simulink model "test_pid_exact_3"  (R2021a)
settings: Solver=VariableStepAuto  StartTime=0.0  StopTime=2000  FixedStep=10  RelTol=1e-3
StopFcn:
  | out1=out;
values from neighbouring files (symbols this model uses):
  Force_Vectors = [Force_Vectors;normal_vector]    [ellip_force_test.m]    (also in initial_sim.m = Force_Vectors'; initial_sim2.m = Force_Vectors'; multi_sim.m = Force_Vectors'; multi_sim2.m = Force_Vectors')
  Km_d = inputArg(2)    [cost_pwpf_dis.m]
  max_f = 100000    [initial_sim.m]    (also in initial_sim2.m = 10)
  max_F_available = max_F_available*0.7    [initial_sim.m]    (also in initial_sim2.m)
  max_M_available = max_M_available*0.7    [initial_sim.m]    (also in initial_sim2.m; multi_sim.m; multi_sim2.m)
  mee_0 = oe2mee([a_0 e_0 incl_0 omega_0 RA_0 theta_0],p.mu)'    [Sample_OT.m]    (also in initial_sim.m = oe2mee(oe_0,params.mu)'; initial_sim2.m = oe2mee(oe_0,params.mu))
  Moment_Vectors = [Moment_Vectors;cross([x y z],normal_vector)]    [ellip_force_test.m]    (also in initial_sim.m = Moment_Vectors'; initial_sim2.m = Moment_Vectors'; multi_sim.m = Moment_Vectors'; multi_sim2.m = Moment_Vectors')
  N_sat = length(azimuths)    [ellip_force_test.m]    (also in initial_sim.m = 30; initial_sim2.m = 25; multi_sim.m = sim_data.N_sat; multi_sim2.m = sim_data.N_sat)
  out = (1+u).*cost_repo_limt.*(cost_repo).^2    [cost.m]    (also in cost2.m)
  params = 0    [Combo_OT.m]
  scale = length_real/(max(x)-min(x))    [model3d_maker.m]
  Tm_d = inputArg(1)    [cost_pwpf_dis.m]
  u_off = inputArg(4)    [cost_pwpf.m]    (also in cost_pwpf_dis.m)
  u_on = h+u_off    [cost_pwpf.m]    (also in cost_pwpf_dis.m)
undefined symbols (not defined in the file or in its folder): c_rad2deg, min_on_off_time, sample_time
libraries: pid_lib x8, simulink x3, shared6dof x1
settings Model: Creator=Mehdi  LastModifiedBy=Mehdi
settings SolverCC: ZeroCrossAlgorithm=Adaptive  AlgebraicLoopSolver=TrustRegion
settings DebuggingCC: IgnoredZcDiagnostic=none  SFMachineParentedDataDiag=warning

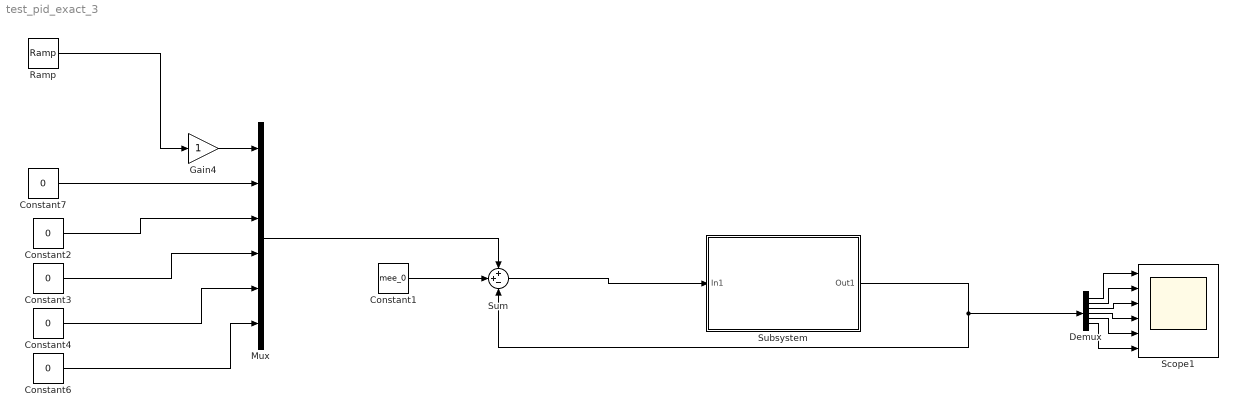
== system test_pid_exact_3 ==
  Constant1 : Constant  Value=mee_0
  Constant{2..4,6..7} (5 alike) : Constant  Value=0
  Demux : Demux  Outputs=6
  Gain4 : Gain
  Mux : Mux  Inputs=6
  Ramp : simulink/Sources/Ramp  slope=-40  start=1  InitialOutput=0
  Scope1 : Scope  NumInputPorts=6
  Subsystem : Subsystem
  Sum : Sum  Inputs=++-
  wires:
  Subsystem/1(Out1) -> Sum/3, Demux/1
  Demux/5 -> Scope1/5
  Demux/4 -> Scope1/4
  Demux/6 -> Scope1/6
  Demux/3 -> Scope1/3
  Demux/2 -> Scope1/2
  Demux/1 -> Scope1/1
  Constant1/1 -> Sum/2
  Constant7/1 -> Mux/2
  Constant2/1 -> Mux/3
  Constant3/1 -> Mux/4
  Constant4/1 -> Mux/5
  Sum/1 -> Subsystem/1(In1)
  Mux/1 -> Sum/1
  Constant6/1 -> Mux/6
  Ramp/1 -> Gain4/1
  Gain4/1 -> Mux/1

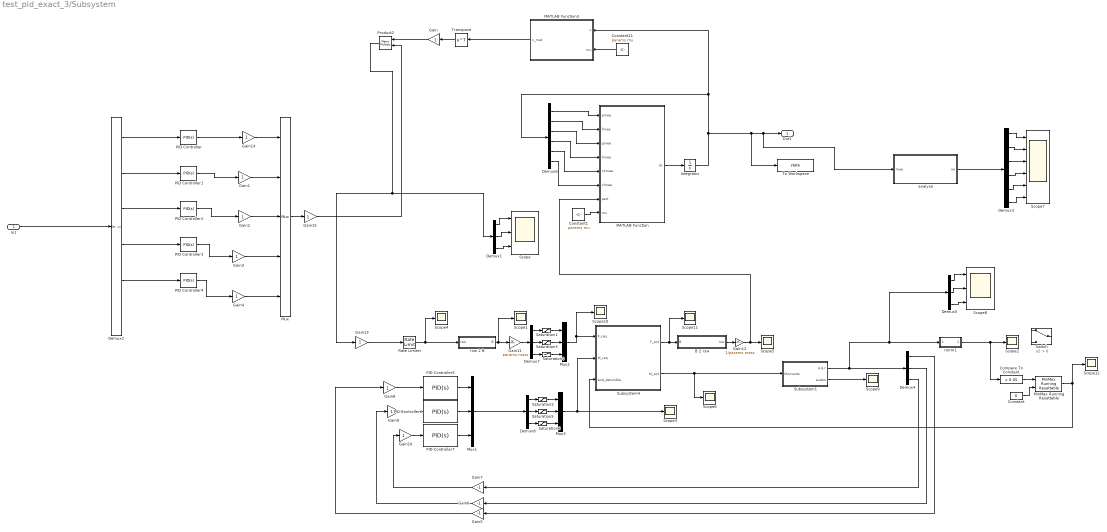
== system test_pid_exact_3/Subsystem ==
  In1 : Inport
  B 2 rsw : Subsystem
  Compare To Constant : simulink/Logic and Bit Operations/Compare To Constant  relop=<  const=0.05  OutDataTypeStr=boolean
  Constant : Constant  Value=0
  Constant1 : Constant  Value=params.mu
  Constant11 : Constant  Value=params.mu
  Demux{1,4..5,7..8} (5 alike) : Demux  Outputs=3
  Demux2 : Demux  Outputs=6
  Demux3 : Demux  Outputs=6
  Demux6 : Demux  Outputs=6
  Gain{,1..4,8..10,13..15} (11 alike) : Gain
  Gain11 : Gain  Gain=params.mass
  Gain12 : Gain  Gain=1/params.mass
  Gain5 : Gain  Gain=-1
  Gain6 : Gain  Gain=-1
  Gain7 : Gain  Gain=-1
  Integrator : Integrator  InitialCondition=mee_0
  MATLAB Function : MATLAB Function  TreatAsAtomicUnit=on
  MATLAB Function3 : MATLAB Function  TreatAsAtomicUnit=on
  MinMax Running Resettable : simulink/Math Operations/MinMax Running Resettable  Function=max  vinit=0.0
  Mux : Mux  Inputs=5
  Mux1 : Mux  Inputs=3
  Mux2 : Mux  Inputs=3
  Mux3 : Mux  Inputs=3
  PID Controller : pid_lib/PID Controller  Controller=PID  Form=Parallel  TimeDomain=Continuous-time  UseExternalTs=off  SampleTime=-1  IntegratorMethod=Forward Euler  FilterMethod=Forward Euler  ControllerParametersSource=internal  P=7.46892494212969e-17  I=7.69051114073229e-19  D=-6.40319929036286e-17  UseFilter=on  N=1.16643643332651  TunerSelectOption=Transfer Function Based (PID Tuner App)  InitialConditionSource=internal  InitialConditionForIntegrator=0  InitialConditionForFilter=0  DifferentiatorICPrevScaledInput=0  ExternalReset=none  TrackingMode=off  Kt=1  LimitOutput=off  SatLimitsSource=internal  UpperSaturationLimit=inf  LowerSaturationLimit=-inf  LinearizeAsGain=on  AntiWindupMode=none  Kb=1  POutMin=[]  POutMax=[]  IOutMin=[]  IOutMax=[]  DOutMin=[]  DOutMax=[]  NOutMin=[]  NOutMax=[]  SumOutMin=[]  SumOutMax=[]  SaturationOutMin=[]  SaturationOutMax=[]  PParamMin=[]  PParamMax=[]  IParamMin=[]  IParamMax=[]  DParamMin=[]  DParamMax=[]  NParamMin=[]  NParamMax=[]  KbParamMin=[]  KbParamMax=[]  KtParamMin=[]  KtParamMax=[]  KbOutMin=[]  KbOutMax=[]  KtOutMin=[]  KtOutMax=[]  IntegratorOutMin=[]  IntegratorOutMax=[]  FilterOutMin=[]  FilterOutMax=[]  SumI1OutMin=[]  SumI1OutMax=[]  SumI2OutMin=[]  SumI2OutMax=[]  SumI3OutMin=[]  SumI3OutMax=[]  SumI4OutMin=[]  SumI4OutMax=[]  SumDOutMin=[]  SumDOutMax=[]  DifferentiatorOutMin=[]  DifferentiatorOutMax=[]  FilterDiffOutCoefMin=[]  FilterDiffOutCoefMax=[]  ReciprocalOutMin=[]  ReciprocalOutMax=[]  SumDenOutMin=[]  SumDenOutMax=[]  SumNumOutMin=[]  SumNumOutMax=[]  DivideOutMin=[]  DivideOutMax=[]  UdiffTsProdOutMin=[]  UdiffTsProdOutMax=[]  NTsProdOutMin=[]  NTsProdOutMax=[]  UintegralTsProdOutMin=[]  UintegralTsProdOutMax=[]  UngainTsProdOutMin=[]  UngainTsProdOutMax=[]  IntegratorContinuousStateAttributes=''  IntegratorStateMustResolveToSignalObject=off  IntegratorRTWStateStorageClass=Auto  FilterContinuousStateAttributes=''  FilterStateMustResolveToSignalObject=off  FilterRTWStateStorageClass=Auto  ParallelPVariant=InternalParameters  IdealPVariant=Disabled  IVariant=InternalParameters  DVariant=InternalParameters  IntegratorVariant=Continuous  SatVariant=Disabled  AWVariant=Passthrough  PCopyVariant=Disabled  TRVariant=Disabled  FdbkBlocksVariant=Forward  IdealPFdbkVariant=Disabled  SatFdbkVariant=Disabled  DerivativeFilterVariant=ContFilter  NVariant=InternalParameters  NCopyVariant=Disabled  FilterICVariant=InternalICsFilter  IntegratorICVariant=InternalICs  ExternalResetVariant=Disabled  TRSumVariant=Passthrough  SumFdbkVariant=Disabled  SumVariant=Sum_PID  TsampFilterVariant=InternalTs  TsampNgainVariant=Passthrough  TsampIntegralVariant=Passthrough  ExternalSaturationOutDataTypeStr=Inherit: Same as second input
  PID Controller1 : pid_lib/PID Controller  Controller=PID  Form=Parallel  TimeDomain=Continuous-time  UseExternalTs=off  SampleTime=-1  IntegratorMethod=Forward Euler  FilterMethod=Forward Euler  ControllerParametersSource=internal  P=0.0771610720825314  I=1.00385329612141e-05  D=-57.2451341733765  UseFilter=on  N=0.000145942090581238  TunerSelectOption=Transfer Function Based (PID Tuner App)  InitialConditionSource=internal  InitialConditionForIntegrator=0  InitialConditionForFilter=0  DifferentiatorICPrevScaledInput=0  ExternalReset=none  TrackingMode=off  Kt=1  LimitOutput=off  SatLimitsSource=internal  UpperSaturationLimit=inf  LowerSaturationLimit=-inf  LinearizeAsGain=on  AntiWindupMode=none  Kb=1  POutMin=[]  POutMax=[]  IOutMin=[]  IOutMax=[]  DOutMin=[]  DOutMax=[]  NOutMin=[]  NOutMax=[]  SumOutMin=[]  SumOutMax=[]  SaturationOutMin=[]  SaturationOutMax=[]  PParamMin=[]  PParamMax=[]  IParamMin=[]  IParamMax=[]  DParamMin=[]  DParamMax=[]  NParamMin=[]  NParamMax=[]  KbParamMin=[]  KbParamMax=[]  KtParamMin=[]  KtParamMax=[]  KbOutMin=[]  KbOutMax=[]  KtOutMin=[]  KtOutMax=[]  IntegratorOutMin=[]  IntegratorOutMax=[]  FilterOutMin=[]  FilterOutMax=[]  SumI1OutMin=[]  SumI1OutMax=[]  SumI2OutMin=[]  SumI2OutMax=[]  SumI3OutMin=[]  SumI3OutMax=[]  SumI4OutMin=[]  SumI4OutMax=[]  SumDOutMin=[]  SumDOutMax=[]  DifferentiatorOutMin=[]  DifferentiatorOutMax=[]  FilterDiffOutCoefMin=[]  FilterDiffOutCoefMax=[]  ReciprocalOutMin=[]  ReciprocalOutMax=[]  SumDenOutMin=[]  SumDenOutMax=[]  SumNumOutMin=[]  SumNumOutMax=[]  DivideOutMin=[]  DivideOutMax=[]  UdiffTsProdOutMin=[]  UdiffTsProdOutMax=[]  NTsProdOutMin=[]  NTsProdOutMax=[]  UintegralTsProdOutMin=[]  UintegralTsProdOutMax=[]  UngainTsProdOutMin=[]  UngainTsProdOutMax=[]  IntegratorContinuousStateAttributes=''  IntegratorStateMustResolveToSignalObject=off  IntegratorRTWStateStorageClass=Auto  FilterContinuousStateAttributes=''  FilterStateMustResolveToSignalObject=off  FilterRTWStateStorageClass=Auto  ParallelPVariant=InternalParameters  IdealPVariant=Disabled  IVariant=InternalParameters  DVariant=InternalParameters  IntegratorVariant=Continuous  SatVariant=Disabled  AWVariant=Passthrough  PCopyVariant=Disabled  TRVariant=Disabled  FdbkBlocksVariant=Forward  IdealPFdbkVariant=Disabled  SatFdbkVariant=Disabled  DerivativeFilterVariant=ContFilter  NVariant=InternalParameters  NCopyVariant=Disabled  FilterICVariant=InternalICsFilter  IntegratorICVariant=InternalICs  ExternalResetVariant=Disabled  TRSumVariant=Passthrough  SumFdbkVariant=Disabled  SumVariant=Sum_PID  TsampFilterVariant=InternalTs  TsampNgainVariant=Passthrough  TsampIntegralVariant=Passthrough  ExternalSaturationOutDataTypeStr=Inherit: Same as second input
  PID Controller2 : pid_lib/PID Controller  Controller=PID  Form=Parallel  TimeDomain=Continuous-time  UseExternalTs=off  SampleTime=-1  IntegratorMethod=Forward Euler  FilterMethod=Forward Euler  ControllerParametersSource=internal  P=13.6496659854925  I=0.00798827574318409  D=-3629.49576294824  UseFilter=on  N=0.00260459411605955  TunerSelectOption=Transfer Function Based (PID Tuner App)  InitialConditionSource=internal  InitialConditionForIntegrator=0  InitialConditionForFilter=0  DifferentiatorICPrevScaledInput=0  ExternalReset=none  TrackingMode=off  Kt=1  LimitOutput=off  SatLimitsSource=internal  UpperSaturationLimit=inf  LowerSaturationLimit=-inf  LinearizeAsGain=on  AntiWindupMode=none  Kb=1  POutMin=[]  POutMax=[]  IOutMin=[]  IOutMax=[]  DOutMin=[]  DOutMax=[]  NOutMin=[]  NOutMax=[]  SumOutMin=[]  SumOutMax=[]  SaturationOutMin=[]  SaturationOutMax=[]  PParamMin=[]  PParamMax=[]  IParamMin=[]  IParamMax=[]  DParamMin=[]  DParamMax=[]  NParamMin=[]  NParamMax=[]  KbParamMin=[]  KbParamMax=[]  KtParamMin=[]  KtParamMax=[]  KbOutMin=[]  KbOutMax=[]  KtOutMin=[]  KtOutMax=[]  IntegratorOutMin=[]  IntegratorOutMax=[]  FilterOutMin=[]  FilterOutMax=[]  SumI1OutMin=[]  SumI1OutMax=[]  SumI2OutMin=[]  SumI2OutMax=[]  SumI3OutMin=[]  SumI3OutMax=[]  SumI4OutMin=[]  SumI4OutMax=[]  SumDOutMin=[]  SumDOutMax=[]  DifferentiatorOutMin=[]  DifferentiatorOutMax=[]  FilterDiffOutCoefMin=[]  FilterDiffOutCoefMax=[]  ReciprocalOutMin=[]  ReciprocalOutMax=[]  SumDenOutMin=[]  SumDenOutMax=[]  SumNumOutMin=[]  SumNumOutMax=[]  DivideOutMin=[]  DivideOutMax=[]  UdiffTsProdOutMin=[]  UdiffTsProdOutMax=[]  NTsProdOutMin=[]  NTsProdOutMax=[]  UintegralTsProdOutMin=[]  UintegralTsProdOutMax=[]  UngainTsProdOutMin=[]  UngainTsProdOutMax=[]  IntegratorContinuousStateAttributes=''  IntegratorStateMustResolveToSignalObject=off  IntegratorRTWStateStorageClass=Auto  FilterContinuousStateAttributes=''  FilterStateMustResolveToSignalObject=off  FilterRTWStateStorageClass=Auto  ParallelPVariant=InternalParameters  IdealPVariant=Disabled  IVariant=InternalParameters  DVariant=InternalParameters  IntegratorVariant=Continuous  SatVariant=Disabled  AWVariant=Passthrough  PCopyVariant=Disabled  TRVariant=Disabled  FdbkBlocksVariant=Forward  IdealPFdbkVariant=Disabled  SatFdbkVariant=Disabled  DerivativeFilterVariant=ContFilter  NVariant=InternalParameters  NCopyVariant=Disabled  FilterICVariant=InternalICsFilter  IntegratorICVariant=InternalICs  ExternalResetVariant=Disabled  TRSumVariant=Passthrough  SumFdbkVariant=Disabled  SumVariant=Sum_PID  TsampFilterVariant=InternalTs  TsampNgainVariant=Passthrough  TsampIntegralVariant=Passthrough  ExternalSaturationOutDataTypeStr=Inherit: Same as second input
  PID Controller3 : pid_lib/PID Controller  Controller=PID  Form=Parallel  TimeDomain=Continuous-time  UseExternalTs=off  SampleTime=-1  IntegratorMethod=Forward Euler  FilterMethod=Forward Euler  ControllerParametersSource=internal  P=1671.28261526635  I=9.96877148902592  D=-11671.5713850813  UseFilter=on  N=0.0760436593196284  TunerSelectOption=Transfer Function Based (PID Tuner App)  InitialConditionSource=internal  InitialConditionForIntegrator=0  InitialConditionForFilter=0  DifferentiatorICPrevScaledInput=0  ExternalReset=none  TrackingMode=off  Kt=1  LimitOutput=off  SatLimitsSource=internal  UpperSaturationLimit=inf  LowerSaturationLimit=-inf  LinearizeAsGain=on  AntiWindupMode=none  Kb=1  POutMin=[]  POutMax=[]  IOutMin=[]  IOutMax=[]  DOutMin=[]  DOutMax=[]  NOutMin=[]  NOutMax=[]  SumOutMin=[]  SumOutMax=[]  SaturationOutMin=[]  SaturationOutMax=[]  PParamMin=[]  PParamMax=[]  IParamMin=[]  IParamMax=[]  DParamMin=[]  DParamMax=[]  NParamMin=[]  NParamMax=[]  KbParamMin=[]  KbParamMax=[]  KtParamMin=[]  KtParamMax=[]  KbOutMin=[]  KbOutMax=[]  KtOutMin=[]  KtOutMax=[]  IntegratorOutMin=[]  IntegratorOutMax=[]  FilterOutMin=[]  FilterOutMax=[]  SumI1OutMin=[]  SumI1OutMax=[]  SumI2OutMin=[]  SumI2OutMax=[]  SumI3OutMin=[]  SumI3OutMax=[]  SumI4OutMin=[]  SumI4OutMax=[]  SumDOutMin=[]  SumDOutMax=[]  DifferentiatorOutMin=[]  DifferentiatorOutMax=[]  FilterDiffOutCoefMin=[]  FilterDiffOutCoefMax=[]  ReciprocalOutMin=[]  ReciprocalOutMax=[]  SumDenOutMin=[]  SumDenOutMax=[]  SumNumOutMin=[]  SumNumOutMax=[]  DivideOutMin=[]  DivideOutMax=[]  UdiffTsProdOutMin=[]  UdiffTsProdOutMax=[]  NTsProdOutMin=[]  NTsProdOutMax=[]  UintegralTsProdOutMin=[]  UintegralTsProdOutMax=[]  UngainTsProdOutMin=[]  UngainTsProdOutMax=[]  IntegratorContinuousStateAttributes=''  IntegratorStateMustResolveToSignalObject=off  IntegratorRTWStateStorageClass=Auto  FilterContinuousStateAttributes=''  FilterStateMustResolveToSignalObject=off  FilterRTWStateStorageClass=Auto  ParallelPVariant=InternalParameters  IdealPVariant=Disabled  IVariant=InternalParameters  DVariant=InternalParameters  IntegratorVariant=Continuous  SatVariant=Disabled  AWVariant=Passthrough  PCopyVariant=Disabled  TRVariant=Disabled  FdbkBlocksVariant=Forward  IdealPFdbkVariant=Disabled  SatFdbkVariant=Disabled  DerivativeFilterVariant=ContFilter  NVariant=InternalParameters  NCopyVariant=Disabled  FilterICVariant=InternalICsFilter  IntegratorICVariant=InternalICs  ExternalResetVariant=Disabled  TRSumVariant=Passthrough  SumFdbkVariant=Disabled  SumVariant=Sum_PID  TsampFilterVariant=InternalTs  TsampNgainVariant=Passthrough  TsampIntegralVariant=Passthrough  ExternalSaturationOutDataTypeStr=Inherit: Same as second input
  PID Controller4 : pid_lib/PID Controller  Controller=PID  Form=Parallel  TimeDomain=Continuous-time  UseExternalTs=off  SampleTime=-1  IntegratorMethod=Forward Euler  FilterMethod=Forward Euler  ControllerParametersSource=internal  P=479.365255304021  I=32.91768970317  D=214.700467675545  UseFilter=on  N=13.9469234742288  TunerSelectOption=Transfer Function Based (PID Tuner App)  InitialConditionSource=internal  InitialConditionForIntegrator=0  InitialConditionForFilter=0  DifferentiatorICPrevScaledInput=0  ExternalReset=none  TrackingMode=off  Kt=1  LimitOutput=off  SatLimitsSource=internal  UpperSaturationLimit=inf  LowerSaturationLimit=-inf  LinearizeAsGain=on  AntiWindupMode=none  Kb=1  POutMin=[]  POutMax=[]  IOutMin=[]  IOutMax=[]  DOutMin=[]  DOutMax=[]  NOutMin=[]  NOutMax=[]  SumOutMin=[]  SumOutMax=[]  SaturationOutMin=[]  SaturationOutMax=[]  PParamMin=[]  PParamMax=[]  IParamMin=[]  IParamMax=[]  DParamMin=[]  DParamMax=[]  NParamMin=[]  NParamMax=[]  KbParamMin=[]  KbParamMax=[]  KtParamMin=[]  KtParamMax=[]  KbOutMin=[]  KbOutMax=[]  KtOutMin=[]  KtOutMax=[]  IntegratorOutMin=[]  IntegratorOutMax=[]  FilterOutMin=[]  FilterOutMax=[]  SumI1OutMin=[]  SumI1OutMax=[]  SumI2OutMin=[]  SumI2OutMax=[]  SumI3OutMin=[]  SumI3OutMax=[]  SumI4OutMin=[]  SumI4OutMax=[]  SumDOutMin=[]  SumDOutMax=[]  DifferentiatorOutMin=[]  DifferentiatorOutMax=[]  FilterDiffOutCoefMin=[]  FilterDiffOutCoefMax=[]  ReciprocalOutMin=[]  ReciprocalOutMax=[]  SumDenOutMin=[]  SumDenOutMax=[]  SumNumOutMin=[]  SumNumOutMax=[]  DivideOutMin=[]  DivideOutMax=[]  UdiffTsProdOutMin=[]  UdiffTsProdOutMax=[]  NTsProdOutMin=[]  NTsProdOutMax=[]  UintegralTsProdOutMin=[]  UintegralTsProdOutMax=[]  UngainTsProdOutMin=[]  UngainTsProdOutMax=[]  IntegratorContinuousStateAttributes=''  IntegratorStateMustResolveToSignalObject=off  IntegratorRTWStateStorageClass=Auto  FilterContinuousStateAttributes=''  FilterStateMustResolveToSignalObject=off  FilterRTWStateStorageClass=Auto  ParallelPVariant=InternalParameters  IdealPVariant=Disabled  IVariant=InternalParameters  DVariant=InternalParameters  IntegratorVariant=Continuous  SatVariant=Disabled  AWVariant=Passthrough  PCopyVariant=Disabled  TRVariant=Disabled  FdbkBlocksVariant=Forward  IdealPFdbkVariant=Disabled  SatFdbkVariant=Disabled  DerivativeFilterVariant=ContFilter  NVariant=InternalParameters  NCopyVariant=Disabled  FilterICVariant=InternalICsFilter  IntegratorICVariant=InternalICs  ExternalResetVariant=Disabled  TRSumVariant=Passthrough  SumFdbkVariant=Disabled  SumVariant=Sum_PID  TsampFilterVariant=InternalTs  TsampNgainVariant=Passthrough  TsampIntegralVariant=Passthrough  ExternalSaturationOutDataTypeStr=Inherit: Same as second input
  PID Controller5 : pid_lib/PID Controller  Controller=PID  Form=Parallel  TimeDomain=Continuous-time  UseExternalTs=off  SampleTime=-1  IntegratorMethod=Forward Euler  FilterMethod=Forward Euler  ControllerParametersSource=internal  P=493.267124009933  I=0.0943532881280952  D=-103949.358808414  UseFilter=on  N=0.00172044274974478  TunerSelectOption=Transfer Function Based (PID Tuner App)  InitialConditionSource=internal  InitialConditionForIntegrator=0  InitialConditionForFilter=0  DifferentiatorICPrevScaledInput=0  ExternalReset=none  TrackingMode=off  Kt=1  LimitOutput=off  SatLimitsSource=internal  UpperSaturationLimit=inf  LowerSaturationLimit=-inf  LinearizeAsGain=on  AntiWindupMode=none  Kb=1  POutMin=[]  POutMax=[]  IOutMin=[]  IOutMax=[]  DOutMin=[]  DOutMax=[]  NOutMin=[]  NOutMax=[]  SumOutMin=[]  SumOutMax=[]  SaturationOutMin=[]  SaturationOutMax=[]  PParamMin=[]  PParamMax=[]  IParamMin=[]  IParamMax=[]  DParamMin=[]  DParamMax=[]  NParamMin=[]  NParamMax=[]  KbParamMin=[]  KbParamMax=[]  KtParamMin=[]  KtParamMax=[]  KbOutMin=[]  KbOutMax=[]  KtOutMin=[]  KtOutMax=[]  IntegratorOutMin=[]  IntegratorOutMax=[]  FilterOutMin=[]  FilterOutMax=[]  SumI1OutMin=[]  SumI1OutMax=[]  SumI2OutMin=[]  SumI2OutMax=[]  SumI3OutMin=[]  SumI3OutMax=[]  SumI4OutMin=[]  SumI4OutMax=[]  SumDOutMin=[]  SumDOutMax=[]  DifferentiatorOutMin=[]  DifferentiatorOutMax=[]  FilterDiffOutCoefMin=[]  FilterDiffOutCoefMax=[]  ReciprocalOutMin=[]  ReciprocalOutMax=[]  SumDenOutMin=[]  SumDenOutMax=[]  SumNumOutMin=[]  SumNumOutMax=[]  DivideOutMin=[]  DivideOutMax=[]  UdiffTsProdOutMin=[]  UdiffTsProdOutMax=[]  NTsProdOutMin=[]  NTsProdOutMax=[]  UintegralTsProdOutMin=[]  UintegralTsProdOutMax=[]  UngainTsProdOutMin=[]  UngainTsProdOutMax=[]  IntegratorContinuousStateAttributes=''  IntegratorStateMustResolveToSignalObject=off  IntegratorRTWStateStorageClass=Auto  FilterContinuousStateAttributes=''  FilterStateMustResolveToSignalObject=off  FilterRTWStateStorageClass=Auto  ParallelPVariant=InternalParameters  IdealPVariant=Disabled  IVariant=InternalParameters  DVariant=InternalParameters  IntegratorVariant=Continuous  SatVariant=Disabled  AWVariant=Passthrough  PCopyVariant=Disabled  TRVariant=Disabled  FdbkBlocksVariant=Forward  IdealPFdbkVariant=Disabled  SatFdbkVariant=Disabled  DerivativeFilterVariant=ContFilter  NVariant=InternalParameters  NCopyVariant=Disabled  FilterICVariant=InternalICsFilter  IntegratorICVariant=InternalICs  ExternalResetVariant=Disabled  TRSumVariant=Passthrough  SumFdbkVariant=Disabled  SumVariant=Sum_PID  TsampFilterVariant=InternalTs  TsampNgainVariant=Passthrough  TsampIntegralVariant=Passthrough  ExternalSaturationOutDataTypeStr=Inherit: Same as second input
  PID Controller6 : pid_lib/PID Controller  Controller=PID  Form=Parallel  TimeDomain=Continuous-time  UseExternalTs=off  SampleTime=-1  IntegratorMethod=Forward Euler  FilterMethod=Forward Euler  ControllerParametersSource=internal  P=493.267124009933  I=0.0943532881280952  D=-103949.358808414  UseFilter=on  N=0.00172044274974478  TunerSelectOption=Transfer Function Based (PID Tuner App)  InitialConditionSource=internal  InitialConditionForIntegrator=0  InitialConditionForFilter=0  DifferentiatorICPrevScaledInput=0  ExternalReset=none  TrackingMode=off  Kt=1  LimitOutput=off  SatLimitsSource=internal  UpperSaturationLimit=inf  LowerSaturationLimit=-inf  LinearizeAsGain=on  AntiWindupMode=none  Kb=1  POutMin=[]  POutMax=[]  IOutMin=[]  IOutMax=[]  DOutMin=[]  DOutMax=[]  NOutMin=[]  NOutMax=[]  SumOutMin=[]  SumOutMax=[]  SaturationOutMin=[]  SaturationOutMax=[]  PParamMin=[]  PParamMax=[]  IParamMin=[]  IParamMax=[]  DParamMin=[]  DParamMax=[]  NParamMin=[]  NParamMax=[]  KbParamMin=[]  KbParamMax=[]  KtParamMin=[]  KtParamMax=[]  KbOutMin=[]  KbOutMax=[]  KtOutMin=[]  KtOutMax=[]  IntegratorOutMin=[]  IntegratorOutMax=[]  FilterOutMin=[]  FilterOutMax=[]  SumI1OutMin=[]  SumI1OutMax=[]  SumI2OutMin=[]  SumI2OutMax=[]  SumI3OutMin=[]  SumI3OutMax=[]  SumI4OutMin=[]  SumI4OutMax=[]  SumDOutMin=[]  SumDOutMax=[]  DifferentiatorOutMin=[]  DifferentiatorOutMax=[]  FilterDiffOutCoefMin=[]  FilterDiffOutCoefMax=[]  ReciprocalOutMin=[]  ReciprocalOutMax=[]  SumDenOutMin=[]  SumDenOutMax=[]  SumNumOutMin=[]  SumNumOutMax=[]  DivideOutMin=[]  DivideOutMax=[]  UdiffTsProdOutMin=[]  UdiffTsProdOutMax=[]  NTsProdOutMin=[]  NTsProdOutMax=[]  UintegralTsProdOutMin=[]  UintegralTsProdOutMax=[]  UngainTsProdOutMin=[]  UngainTsProdOutMax=[]  IntegratorContinuousStateAttributes=''  IntegratorStateMustResolveToSignalObject=off  IntegratorRTWStateStorageClass=Auto  FilterContinuousStateAttributes=''  FilterStateMustResolveToSignalObject=off  FilterRTWStateStorageClass=Auto  ParallelPVariant=InternalParameters  IdealPVariant=Disabled  IVariant=InternalParameters  DVariant=InternalParameters  IntegratorVariant=Continuous  SatVariant=Disabled  AWVariant=Passthrough  PCopyVariant=Disabled  TRVariant=Disabled  FdbkBlocksVariant=Forward  IdealPFdbkVariant=Disabled  SatFdbkVariant=Disabled  DerivativeFilterVariant=ContFilter  NVariant=InternalParameters  NCopyVariant=Disabled  FilterICVariant=InternalICsFilter  IntegratorICVariant=InternalICs  ExternalResetVariant=Disabled  TRSumVariant=Passthrough  SumFdbkVariant=Disabled  SumVariant=Sum_PID  TsampFilterVariant=InternalTs  TsampNgainVariant=Passthrough  TsampIntegralVariant=Passthrough  ExternalSaturationOutDataTypeStr=Inherit: Same as second input
  PID Controller7 : pid_lib/PID Controller  Controller=PID  Form=Parallel  TimeDomain=Continuous-time  UseExternalTs=off  SampleTime=-1  IntegratorMethod=Forward Euler  FilterMethod=Forward Euler  ControllerParametersSource=internal  P=493.267124009933  I=0.0943532881280952  D=-103949.358808414  UseFilter=on  N=0.00172044274974478  TunerSelectOption=Transfer Function Based (PID Tuner App)  InitialConditionSource=internal  InitialConditionForIntegrator=0  InitialConditionForFilter=0  DifferentiatorICPrevScaledInput=0  ExternalReset=none  TrackingMode=off  Kt=1  LimitOutput=off  SatLimitsSource=internal  UpperSaturationLimit=inf  LowerSaturationLimit=-inf  LinearizeAsGain=on  AntiWindupMode=none  Kb=1  POutMin=[]  POutMax=[]  IOutMin=[]  IOutMax=[]  DOutMin=[]  DOutMax=[]  NOutMin=[]  NOutMax=[]  SumOutMin=[]  SumOutMax=[]  SaturationOutMin=[]  SaturationOutMax=[]  PParamMin=[]  PParamMax=[]  IParamMin=[]  IParamMax=[]  DParamMin=[]  DParamMax=[]  NParamMin=[]  NParamMax=[]  KbParamMin=[]  KbParamMax=[]  KtParamMin=[]  KtParamMax=[]  KbOutMin=[]  KbOutMax=[]  KtOutMin=[]  KtOutMax=[]  IntegratorOutMin=[]  IntegratorOutMax=[]  FilterOutMin=[]  FilterOutMax=[]  SumI1OutMin=[]  SumI1OutMax=[]  SumI2OutMin=[]  SumI2OutMax=[]  SumI3OutMin=[]  SumI3OutMax=[]  SumI4OutMin=[]  SumI4OutMax=[]  SumDOutMin=[]  SumDOutMax=[]  DifferentiatorOutMin=[]  DifferentiatorOutMax=[]  FilterDiffOutCoefMin=[]  FilterDiffOutCoefMax=[]  ReciprocalOutMin=[]  ReciprocalOutMax=[]  SumDenOutMin=[]  SumDenOutMax=[]  SumNumOutMin=[]  SumNumOutMax=[]  DivideOutMin=[]  DivideOutMax=[]  UdiffTsProdOutMin=[]  UdiffTsProdOutMax=[]  NTsProdOutMin=[]  NTsProdOutMax=[]  UintegralTsProdOutMin=[]  UintegralTsProdOutMax=[]  UngainTsProdOutMin=[]  UngainTsProdOutMax=[]  IntegratorContinuousStateAttributes=''  IntegratorStateMustResolveToSignalObject=off  IntegratorRTWStateStorageClass=Auto  FilterContinuousStateAttributes=''  FilterStateMustResolveToSignalObject=off  FilterRTWStateStorageClass=Auto  ParallelPVariant=InternalParameters  IdealPVariant=Disabled  IVariant=InternalParameters  DVariant=InternalParameters  IntegratorVariant=Continuous  SatVariant=Disabled  AWVariant=Passthrough  PCopyVariant=Disabled  TRVariant=Disabled  FdbkBlocksVariant=Forward  IdealPFdbkVariant=Disabled  SatFdbkVariant=Disabled  DerivativeFilterVariant=ContFilter  NVariant=InternalParameters  NCopyVariant=Disabled  FilterICVariant=InternalICsFilter  IntegratorICVariant=InternalICs  ExternalResetVariant=Disabled  TRSumVariant=Passthrough  SumFdbkVariant=Disabled  SumVariant=Sum_PID  TsampFilterVariant=InternalTs  TsampNgainVariant=Passthrough  TsampIntegralVariant=Passthrough  ExternalSaturationOutDataTypeStr=Inherit: Same as second input
  Product2 : Product  Multiplication=Matrix(*)
  Rate Limiter : RateLimiter  RisingSlewLimit=1e-4  FallingSlewLimit=-1e-4  SampleTimeMode=inherited
  Saturation1 : Saturate  UpperLimit=max_F_available(1,1)  LowerLimit=max_F_available(1,2)
  Saturation2 : Saturate  UpperLimit=max_M_available(1,1)  LowerLimit=max_M_available(1,2)
  Saturation3 : Saturate  UpperLimit=max_F_available(2,1)  LowerLimit=max_F_available(2,2)
  Saturation4 : Saturate  UpperLimit=max_F_available(3,1)  LowerLimit=max_F_available(3,2)
  Saturation5 : Saturate  UpperLimit=max_M_available(2,1)  LowerLimit=max_M_available(2,2)
  Saturation6 : Saturate  UpperLimit=max_M_available(3,1)  LowerLimit=max_M_available(3,2)
  Scope : Scope  NumInputPorts=3
  Scope{1..6,9..12} (10 alike) : Scope
  Scope7 : Scope  NumInputPorts=6
  Scope8 : Scope  NumInputPorts=3
  Subsystem1 : Subsystem
  Subsystem4 : Subsystem
  Switch : Switch  Criteria=u2 > Threshold
  To Workspace : ToWorkspace  VariableName=state  SaveFormat=Timeseries  SampleTime=-1
  Transpose : Math  Operator=transpose  SaturateOnIntegerOverflow=on
  analyse : Subsystem
  norm1 : Subsystem
  rsw 2 B : Subsystem
  Out1 : Outport
  wires:
  Demux6/2 -> MATLAB Function/2(fmee)
  Demux6/1 -> MATLAB Function/1(pmee)
  Demux6/3 -> MATLAB Function/3(gmee)
  Demux6/4 -> MATLAB Function/4(hmee)
  Demux6/5 -> MATLAB Function/5(xkmee)
  Demux6/6 -> MATLAB Function/6(xlmee)
  MATLAB Function/1(dx) -> Integrator/1
  Constant11/1 -> MATLAB Function3/2(mu)
  MATLAB Function3/1(c_mat) -> Transpose/1
  Constant1/1 -> MATLAB Function/8(mu)
  Transpose/1 -> Gain/1
  Gain/1 -> Product2/1
  Demux1/3 -> Scope/3
  Demux1/2 -> Scope/2
  Demux1/1 -> Scope/1
  Demux2/4 -> PID Controller3/1
  Demux2/3 -> PID Controller2/1
  Demux2/5 -> PID Controller4/1
  Demux2/2 -> PID Controller1/1
  Demux2/1 -> PID Controller/1
  In1/1 -> Demux2/1
  Mux/1 -> Gain15/1
  PID Controller/1 -> Gain14/1
  PID Controller1/1 -> Gain1/1
  PID Controller2/1 -> Gain2/1
  PID Controller3/1 -> Gain3/1
  PID Controller4/1 -> Gain4/1
  Gain1/1 -> Mux/2
  Gain2/1 -> Mux/3
  Gain3/1 -> Mux/4
  Gain4/1 -> Mux/5
  Subsystem4/2(M_act) -> Subsystem1/1(Moments), Scope6/1
  Product2/1 -> Gain13/1, Demux1/1
  Demux3/6 -> Scope7/6
  Demux3/1 -> Scope7/1
  Demux3/2 -> Scope7/2
  Demux3/3 -> Scope7/3
  Demux3/4 -> Scope7/4
  Demux3/5 -> Scope7/5
  Integrator/1 -> To Workspace/1, analyse/1(mee), Out1/1, Demux6/1, MATLAB Function3/1(x)
  analyse/1(oe) -> Demux3/1
  Rate Limiter/1 -> rsw 2 B/1(rsw), Scope4/1
  Subsystem4/1(F_act) -> Scope11/1, B 2 rsw/1(B)
  B 2 rsw/1(rsw) -> Gain12/1
  rsw 2 B/1(B) -> Gain11/1, Scope1/1
  Gain8/1 -> PID Controller5/1
  Gain9/1 -> PID Controller6/1
  PID Controller7/1 -> Mux1/3
  Gain7/1 -> Gain10/1
  Demux4/1 -> Gain5/1
  Gain6/1 -> Gain9/1
  Subsystem1/2(eulers) -> Scope9/1
  Demux4/2 -> Gain6/1
  PID Controller5/1 -> Mux1/1
  Demux4/3 -> Gain7/1
  Gain10/1 -> PID Controller7/1
  Gain5/1 -> Gain8/1
  PID Controller6/1 -> Mux1/2
  norm1/1(Out1) -> Scope2/1, Compare To Constant/1
  Subsystem1/1(p,q,r) -> Demux5/1, norm1/1(p,q,r), Demux4/1
  Demux5/1 -> Scope8/1
  Demux5/3 -> Scope8/3
  Demux5/2 -> Scope8/2
  Mux3/1 -> Subsystem4/2(M_req), Scope3/1
  Demux7/1 -> Saturation1/1
  Demux7/2 -> Saturation3/1
  Demux7/3 -> Saturation4/1
  Saturation1/1 -> Mux2/1
  Saturation3/1 -> Mux2/2
  Saturation4/1 -> Mux2/3
  Mux2/1 -> Scope10/1, Subsystem4/1(F_req)
  Demux8/1 -> Saturation2/1
  Demux8/3 -> Saturation6/1
  Saturation6/1 -> Mux3/3
  Saturation5/1 -> Mux3/2
  Demux8/2 -> Saturation5/1
  Saturation2/1 -> Mux3/1
  Mux1/1 -> Demux8/1
  Gain11/1 -> Demux7/1
  Gain12/1 -> Scope5/1, MATLAB Function/7(pert)
  Gain13/1 -> Rate Limiter/1
  Gain14/1 -> Mux/1
  Gain15/1 -> Product2/2
  MinMax Running Resettable/1 -> Scope12/1, Subsystem4/3(end_detumble)
  Compare To Constant/1 -> MinMax Running Resettable/1
  Constant/1 -> MinMax Running Resettable/2

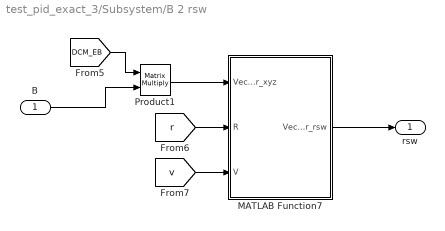
== system test_pid_exact_3/Subsystem/B 2 rsw ==
  B : Inport
  MATLAB Function7 : MATLAB Function  TreatAsAtomicUnit=on
  Product1 : Product  Multiplication=Matrix(*)
  rsw : Outport
  wires:
  Product1/1 -> MATLAB Function7/1(Vector_xyz)
  [v] -> MATLAB Function7/3(V)
  [DCM_EB] -> Product1/1
  [r] -> MATLAB Function7/2(R)
  B/1 -> Product1/2
  MATLAB Function7/1(Vector_rsw) -> rsw/1

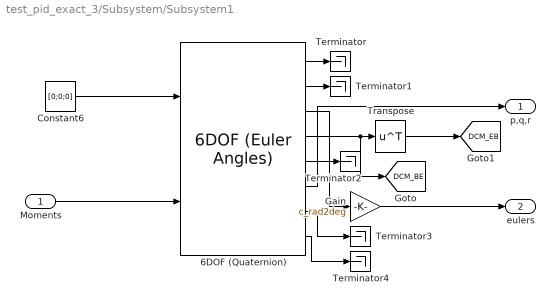
== system test_pid_exact_3/Subsystem/Subsystem1 ==
  Moments : Inport
  6DOF (Quaternion) : shared6dof/6DOF (Euler Angles)  units=Metric (MKS)  mtype=Fixed  rep=Quaternion  xme_0=[0 0 0]  Vm_0=[0 0 0]  eul_0=eul_0  pm_0=pqr_0  mass_0=1.0  mass_e=0.5  mass_f=2.0  inertia=params.Inertia  inertia_e=eye(3)  inertia_f=2*eye(3)  k_quat=1.0  vre_flag=on  abi_flag=off  aMode=0  xme_statename=''  Vm_statename=''  eul_statename=''  quat_statename=''  pm_statename=''  mass_statename=''
      settings: SourceProductBaseCode=AE,PW,DR,MT,UV,VE
  Constant6 : Constant  Value=[0;0;0]
  Gain : Gain  Gain=c_rad2deg
  Terminator{,1..4} (5 alike) : Terminator
  Transpose : Math  Operator=transpose  SaturateOnIntegerOverflow=on
  p,q,r : Outport
  eulers : Outport  Port=2
  tag scope: DCM_BE=global, DCM_EB=global
  wires:
  6DOF (Quaternion)/7 -> Terminator3/1
  Constant6/1 -> 6DOF (Quaternion)/1
  6DOF (Quaternion)/3 -> Gain/1
  6DOF (Quaternion)/1 -> Terminator/1
  6DOF (Quaternion)/6 -> p,q,r/1
  6DOF (Quaternion)/5 -> Terminator2/1
  6DOF (Quaternion)/2 -> Terminator1/1
  Gain/1 -> eulers/1
  6DOF (Quaternion)/4 -> [DCM_BE], Transpose/1
  6DOF (Quaternion)/8 -> Terminator4/1
  Moments/1 -> 6DOF (Quaternion)/2
  Transpose/1 -> [DCM_EB]

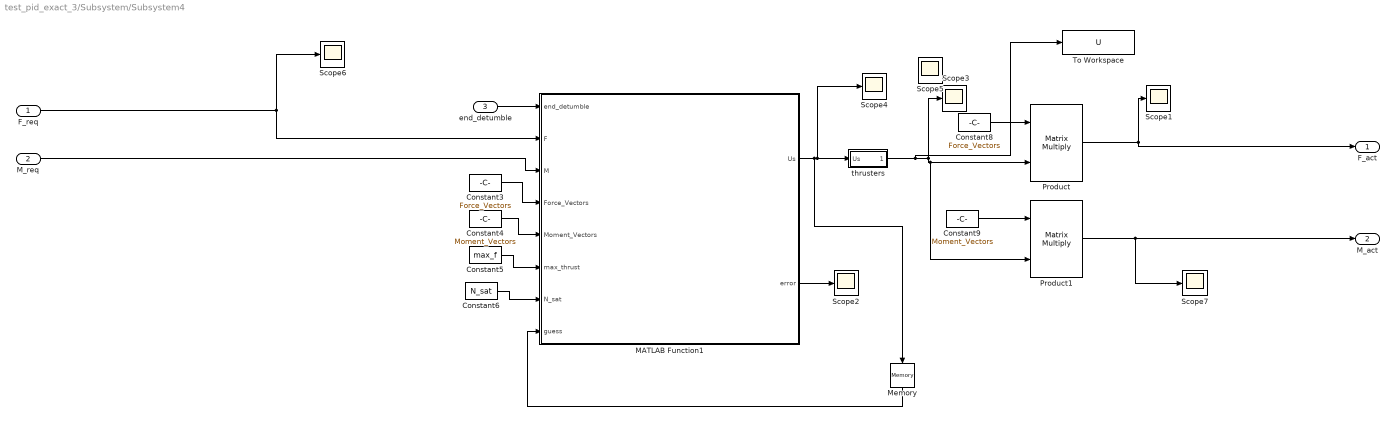
== system test_pid_exact_3/Subsystem/Subsystem4 ==
  F_req : Inport
  M_req : Inport  Port=2
  end_detumble : Inport  Port=3
  Constant3 : Constant  Value=Force_Vectors
  Constant4 : Constant  Value=Moment_Vectors
  Constant5 : Constant  Value=max_f
  Constant6 : Constant  Value=N_sat
  Constant8 : Constant  Value=Force_Vectors
  Constant9 : Constant  Value=Moment_Vectors
  MATLAB Function1 : MATLAB Function  TreatAsAtomicUnit=on
  Memory : Memory  InitialCondition=zeros(N_sat,1)
  Product : Product  Multiplication=Matrix(*)
  Product1 : Product  Multiplication=Matrix(*)
  Scope{1..7} (7 alike) : Scope
  To Workspace : ToWorkspace  VariableName=U  SaveFormat=Timeseries  SampleTime=-1
  thrusters : Subsystem
  F_act : Outport
  M_act : Outport  Port=2
  wires:
  Constant6/1 -> MATLAB Function1/7(N_sat)
  Constant9/1 -> Product1/1
  Memory/1 -> MATLAB Function1/8(guess)
  MATLAB Function1/2(error) -> Scope2/1
  Constant3/1 -> MATLAB Function1/4(Force_Vectors)
  Constant4/1 -> MATLAB Function1/5(Moment_Vectors)
  Product1/1 -> Scope7/1, M_act/1
  Constant8/1 -> Product/1
  Constant5/1 -> MATLAB Function1/6(max_thrust)
  F_req/1 -> MATLAB Function1/2(F), Scope6/1
  M_req/1 -> MATLAB Function1/3(M)
  Product/1 -> F_act/1, Scope1/1
  end_detumble/1 -> MATLAB Function1/1(end_detumble)
  MATLAB Function1/1(Us) -> thrusters/1(Us), Scope4/1, Memory/1
  thrusters/1(U_act) -> To Workspace/1, Product/2, Product1/2, Scope3/1

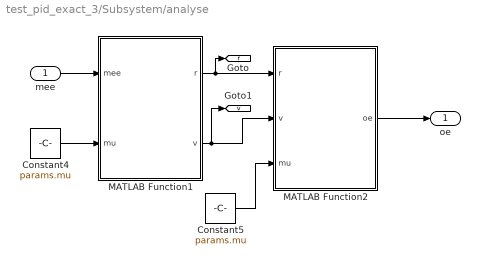
== system test_pid_exact_3/Subsystem/analyse ==
  mee : Inport
  Constant4 : Constant  Value=params.mu
  Constant5 : Constant  Value=params.mu
  MATLAB Function1 : MATLAB Function  TreatAsAtomicUnit=on
  MATLAB Function2 : MATLAB Function  TreatAsAtomicUnit=on
  oe : Outport
  tag scope: r=global, v=global
  wires:
  Constant5/1 -> MATLAB Function2/3(mu)
  Constant4/1 -> MATLAB Function1/2(mu)
  MATLAB Function1/1(r) -> [r], MATLAB Function2/1(r)
  MATLAB Function1/2(v) -> [v], MATLAB Function2/2(v)
  MATLAB Function2/1(oe) -> oe/1
  mee/1 -> MATLAB Function1/1(mee)

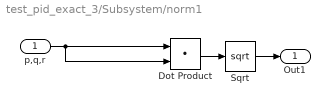
== system test_pid_exact_3/Subsystem/norm1 ==
  p,q,r : Inport
  Dot Product : DotProduct  InputSameDT=on  OutDataTypeStr=Inherit: Inherit via internal rule
  Sqrt : Sqrt  OutputSignalType=real  SaturateOnIntegerOverflow=on
  Out1 : Outport
  wires:
  Dot Product/1 -> Sqrt/1
  p,q,r/1 -> Dot Product/1, Dot Product/2
  Sqrt/1 -> Out1/1

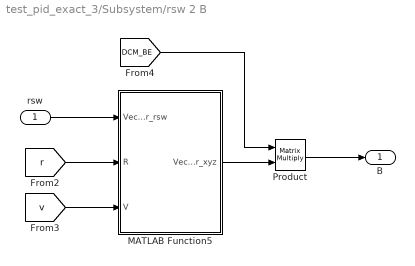
== system test_pid_exact_3/Subsystem/rsw 2 B ==
  rsw : Inport
  MATLAB Function5 : MATLAB Function  TreatAsAtomicUnit=on
  Product : Product  Multiplication=Matrix(*)
  B : Outport
  wires:
  [DCM_BE] -> Product/1
  rsw/1 -> MATLAB Function5/1(Vector_rsw)
  MATLAB Function5/1(Vector_xyz) -> Product/2
  [v] -> MATLAB Function5/3(V)
  [r] -> MATLAB Function5/2(R)
  Product/1 -> B/1

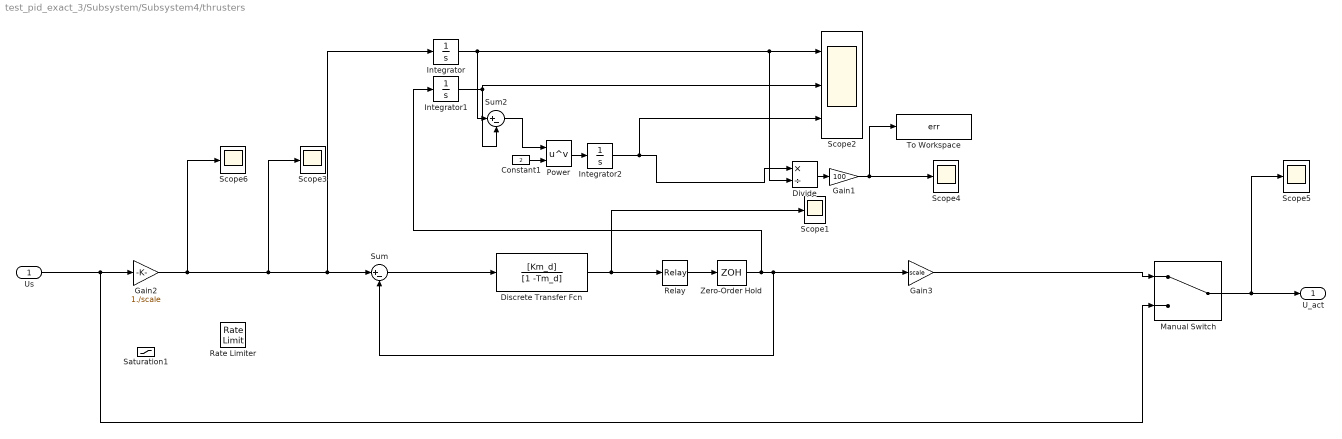
== system test_pid_exact_3/Subsystem/Subsystem4/thrusters ==
  Us : Inport
  Constant1 : Constant  Value=2  VectorParams1D=off
  Discrete Transfer Fcn : DiscreteTransferFcn  Numerator=[Km_d]  Denominator=[1 -Tm_d]  SampleTime=sample_time
  Divide : Product  Inputs=*/
  Gain1 : Gain  Gain=100
  Gain2 : Gain  Gain=1./scale
  Gain3 : Gain  Gain=scale
  Integrator : Integrator
  Integrator1 : Integrator
  Integrator2 : Integrator
  Manual Switch : ManualSwitch
  Power : Math  Operator=pow  SaturateOnIntegerOverflow=on
  Rate Limiter : RateLimiter  RisingSlewLimit=1e-4  FallingSlewLimit=-1e-4  SampleTimeMode=inherited
  Relay : Relay  OnSwitchValue=u_on  OffSwitchValue=u_off  OnOutputValue=Thrust_digital
  Saturation1 : Saturate  UpperLimit=max_f  LowerLimit=0
  Scope{1,3..6} (5 alike) : Scope
  Scope2 : Scope  NumInputPorts=3
  Sum : Sum  Inputs=|+-
  Sum2 : Sum  Inputs=|+-
  To Workspace : ToWorkspace  VariableName=err  SaveFormat=Timeseries  SampleTime=-1
      settings: MaxDataPoints=1
  Zero-Order Hold : ZeroOrderHold  SampleTime=min_on_off_time
  U_act : Outport
  wires:
  Manual Switch/1 -> Scope5/1, U_act/1
  Gain3/1 -> Manual Switch/1
  Divide/1 -> Gain1/1
  Zero-Order Hold/1 -> Integrator1/1, Sum/2, Gain3/1
  Sum/1 -> Discrete Transfer Fcn/1
  Gain1/1 -> To Workspace/1, Scope4/1
  Relay/1 -> Zero-Order Hold/1
  Constant1/1 -> Power/2
  Integrator1/1 -> Sum2/2, Scope2/2
  Discrete Transfer Fcn/1 -> Relay/1, Scope1/1
  Integrator/1 -> Sum2/1, Divide/2, Scope2/1
  Power/1 -> Integrator2/1
  Integrator2/1 -> Scope2/3, Divide/1
  Sum2/1 -> Power/1
  Us/1 -> Gain2/1, Manual Switch/2
  Gain2/1 -> Scope3/1, Integrator/1, Sum/1, Scope6/1

== matlab function test_pid_exact_3/Subsystem/Subsystem4/MATLAB Function1 ==
  data: end_detumble input; F input size=3; Us output; M input size=3; Force_Vectors input; Moment_Vectors input; error output; max_thrust input; N_sat input size=1; guess input
function [Us,error] = cotrol_allocation(end_detumble,F,M,Force_Vectors,Moment_Vectors,max_thrust,N_sat,guess)


if end_detumble==0
    maxIter=10;
    
    % Us=zeros(N_sat,1);
    % Uss=zeros(N_sat,1);
    
    b=[F(1);F(2);F(3);M(1);M(2);M(3)];
    C=[Force_Vectors;Moment_Vectors];
    
    options = optimoptions('lsqnonlin','Algorithm','levenberg-marquardt','MaxIterations',maxIter);
    LB=zeros(N_sat,1);
    UB=max_thrust*ones(N_sat,1);
    % x0=zeros(N_sat,1);
    x0=guess;
    
    % C*x0-b
    
    fun=@(x)(C*x-b);
    
    
    
    [Uss,error]=lsqnonlin(fun,x0,LB,UB,options);
    
    
    
    
    Us=Uss(1:30,1);
    
    %
    % F_out=Force_Vectors*Us;
    % M_out=Moment_Vectors*Us;
    
    
    
    % Us=C*x0-b;
    
    
    % for i=1:N_sat
    %     Us(i)=U1(i);
    % end
    
    % error=0;
    
    
else
    
    maxIter=10;
    
    % Us=zeros(N_sat,1);
    % Uss=zeros(N_sat,1);
    
    b=[F(1);F(2);F(3);0;0;0];
    C=[Force_Vectors;Moment_Vectors];
    
    options = optimoptions('lsqnonlin','Algorithm','levenberg-marquardt','MaxIterations',maxIter);
    LB=zeros(N_sat,1);
    UB=max_thrust*ones(N_sat,1);
    % x0=zeros(N_sat,1);
    x0=guess;
    
    % C*x0-b
    
    fun=@(x)(C*x-b);
    
    
    
    [Uss,error]=lsqnonlin(fun,x0,LB,UB,options);
    
    
    
    
    Us=Uss(1:30,1);
    
    
    
end

end

== matlab function test_pid_exact_3/Subsystem/MATLAB Function ==
  data: pmee input; fmee input; gmee input; hmee input; xkmee input; xlmee input; pert input; dx output; mu input
function dx = path_dynamics(pmee,fmee,gmee,hmee,xkmee,xlmee,pert,mu)


pert_1=pert(1);
pert_2=pert(2);
pert_3=pert(3);
% 
% pmee = x(1);
% fmee = x(2);
% gmee = x(3);
% hmee = x(4);
% xkmee = x(5);
% xlmee = x(6);
% 
% pert_1=u(1);
% pert_2=u(2);
% pert_3=u(3);



%%%%%%% orbital dynamics
smovrp = sqrt(mu / pmee);
tani2s = hmee.^2 + xkmee.^2;
cosl = cos(xlmee);
sinl = sin(xlmee);
wmee = 1.0 + fmee * cosl + gmee * sinl;
ssqrd = 1.0 + tani2s;
meedot_1 = 2.0 * pmee * pert_2 / (wmee * smovrp);
term1 = ((wmee + 1.0) * cosl + fmee) * pert_2;
term2 = (hmee * sinl - xkmee * cosl) * gmee * pert_3;
meedot_2 = (pert_1 * sinl + (term1 - term2) / wmee) / smovrp;
term1 = ((wmee + 1.0) * sinl + gmee) * pert_2;
term2 = (hmee * sinl - xkmee * cosl) * fmee * pert_3;
meedot_3 = (-pert_1 * cosl + (term1 + term2) / wmee) / smovrp;
term1 = ssqrd * pert_3 / (2.0 * wmee * smovrp);
meedot_4 = term1 * cosl;
meedot_5 = term1 * sinl;
meedot_6 = sqrt(mu * pmee) * (wmee / pmee).^2 ...
    + (hmee * sinl - xkmee * cosl) * pert_3/(wmee * smovrp);

%%%%%%%


% dx=[p_dot;q_dot;r_dot;quat0_dot;quat1_dot;quat2_dot;quat3_dot;meedot_1;meedot_2;meedot_3;meedot_4;meedot_5;meedot_6];
dx=[meedot_1;meedot_2;meedot_3;meedot_4;meedot_5;meedot_6];

== matlab function test_pid_exact_3/Subsystem/analyse/MATLAB Function1 ==
  data: mee input; r output; mu input; v output
function [r, v] = mee2rv(mee,mu)

% convert modified equinoctial orbital
% elements to eci position and velocity vectors

% input

%  mu     = gravitational constant (km**3/sec**2)
%  mee(1) = semilatus rectum of orbit (kilometers)
%  mee(2) = f equinoctial element
%  mee(3) = g equinoctial element
%  mee(4) = h equinoctial element
%  mee(5) = k equinoctial element
%  mee(6) = true longitude (radians)

% output

%  r = eci position vector (kilometers)
%  v = eci velocity vector (kilometers/second)

% Orbital Mechanics with MATLAB

%%%%%%%%%%%%%%%%%%%%%%%%%%%%%%%
r = zeros(3, 1);
v = zeros(3, 1);
% unload equinoctial orbital elements

pmee = mee(1);
fmee = mee(2);
gmee = mee(3);
hmee = mee(4);
kmee = mee(5);
lmee = mee(6);

smovrp = sqrt(mu / pmee);

tani2s = hmee^2 + kmee^2;

cosl = cos(lmee);

sinl = sin(lmee);

wmee = 1 + fmee * cosl + gmee * sinl;

radius = pmee / wmee;

hsmks = hmee^2 - kmee^2;

ssqrd = 1 + tani2s;

% compute eci position vector

r(1) = radius * (cosl + hsmks * cosl + 2 * hmee * kmee * sinl) / ssqrd;

r(2) = radius * (sinl - hsmks * sinl + 2 * hmee * kmee * cosl) / ssqrd;

r(3) = 2 * radius * (hmee * sinl - kmee * cosl) / ssqrd;

% compute eci velocity vector

v(1) = - smovrp * (sinl + hsmks * sinl - 2 * hmee * kmee * cosl + gmee ...
       - 2 * fmee * hmee * kmee + hsmks * gmee) / ssqrd;

v(2) = - smovrp * (-cosl + hsmks * cosl + 2 * hmee * kmee * sinl - fmee ...
       + 2 * gmee * hmee * kmee + hsmks * fmee) / ssqrd;

v(3) = 2 * smovrp * (hmee * cosl + kmee * sinl + fmee * hmee ...
       + gmee * kmee) / ssqrd;
   
end

== matlab function test_pid_exact_3/Subsystem/MATLAB Function3 ==
  data: x input; c_mat output; mu input
function c_mat = path_c_mat(x,mu)



pmee = x(1);
fmee = x(2);
gmee = x(3);
hmee = x(4);
xkmee = x(5);
xlmee = x(6);


sin_x=sin(xlmee);
cos_x=cos(xlmee);
sqmuop=sqrt(mu/pmee);
term1=sqmuop* (fmee * cos_x + gmee * sin_x + 1);
term2 = hmee * sin_x - xkmee * cos_x;
term3 =sqmuop * (2 * fmee * cos_x + 2 * gmee * sin_x + 2);
term4 = fmee * cos_x + gmee * sin_x + 2;
term5=hmee^2+xkmee^2+1;


% c_mat=[...
%     0 2*pmee/term1 0
%     sin_x/sqmuop  (fmee + cos_x * term4)/term1  -gmee*term2/term1
%     -cos_x/sqmuop   (gmee + sin_x*term4)/term1   fmee*term2/term1
%     0 0 cos_x*term5/term3
%     0 0 sin_x*term5/term3
%     0 0 term2/term1];


c_mat=[...
    0 2*pmee/term1 0
    sin_x/sqmuop  (fmee + cos_x * term4)/term1  -gmee*term2/term1
    -cos_x/sqmuop   (gmee + sin_x*term4)/term1   fmee*term2/term1
    0 0 cos_x*term5/term3
    0 0 sin_x*term5/term3];




end

== matlab function test_pid_exact_3/Subsystem/analyse/MATLAB Function2 ==
  data: r input; v input; oe output; mu input
function oe = rv2oe (r, v,mu)

% convert eci state vector to six classical orbital
% elements via equinoctial elements

% input

%  mu = central body gravitational constant (km**3/sec**2)
%  r  = eci position vector (kilometers)
%  v  = eci velocity vector (kilometers/second)

% output

%  oev(1) = semimajor axis (kilometers)
%  oev(2) = orbital eccentricity (non-dimensional)
%           (0 <= eccentricity < 1)
%  oev(3) = orbital inclination (radians)
%           (0 <= inclination <= pi)
%  oev(4) = argument of perigee (radians)
%           (0 <= argument of perigee <= 2 pi)
%  oev(5) = right ascension of ascending node (radians)
%           (0 <= raan <= 2 pi)
%  oev(6) = true anomaly (radians)
%           (0 <= true anomaly <= 2 pi)

% Orbital Mechanics with MATLAB
oe=zeros(1,6);
%%%%%%%%%%%%%%%%%%%%%%%%%%%%%%%

pi2 = 2.0 * pi;

% position and velocity magnitude

rmag = norm(r);

vmag = norm(v);

% position unit vector

rhat = r / rmag;

% angular momentum vectors

hv = cross(r, v);

hhat = hv / norm(hv);

% eccentricity vector

vtmp = v / mu;

ecc = cross(vtmp, hv);

ecc = ecc - rhat;

% semimajor axis

sma = 1.0 / (2.0 / rmag - vmag * vmag / mu);

p = hhat(1) / (1.0 + hhat(3));

q = -hhat(2) / (1.0 + hhat(3));

const1 = 1.0 / (1.0 + p * p + q * q);

fhat=zeros(3,1);
ghat=zeros(3,1);

fhat(1) = const1 * (1.0 - p * p + q * q);
fhat(2) = const1 * 2.0 * p * q;
fhat(3) = -const1 * 2.0 * p;

ghat(1) = const1 * 2.0 * p * q;
ghat(2) = const1 * (1.0 + p * p - q * q);
ghat(3) = const1 * 2.0 * q;

h = dot(ecc, ghat);

xk = dot(ecc, fhat);

x1 = dot(r, fhat);

y1 = dot(r, ghat);

% orbital eccentricity

eccm = sqrt(h * h + xk * xk);

% orbital inclination

inc = 2.0 * atan(sqrt(p * p + q * q));

% true longitude

xlambdat = atan3(y1, x1);

% check for equatorial orbit

if (inc > 0.00000001)
    raan = atan3(p, q);
else
    raan = 0.0;
end

% check for circular orbit

if (eccm > 0.00000001)
    argper = mod(atan3(h, xk) - raan, pi2);
else
    argper = 0.0;
end

% true anomaly

tanom = mod(xlambdat - raan - argper, pi2);

% load orbital element vector

oe(1) = sma;
oe(2) = eccm;
oe(3) = inc;
oe(4) = argper;
oe(5) = raan;
oe(6) = tanom;



end

== matlab function test_pid_exact_3/Subsystem/rsw 2 B/MATLAB Function5 ==
  data: Vector_rsw input; R input; Vector_xyz output; V input
function Vector_xyz=rsw2xyz(Vector_rsw,R,V)



e_r=R/norm(R);
h=cross(R,V);
e_w=h/norm(h);
e_s=cross(e_w,e_r);


Vector_xyz=Vector_rsw(1)*e_r+Vector_rsw(2)*e_s+Vector_rsw(3)*e_w;


end

== matlab function test_pid_exact_3/Subsystem/B 2 rsw/MATLAB Function7 ==
  data: Vector_xyz input; R input; Vector_rsw output; V input
function Vector_rsw=xyz2rsw(Vector_xyz,R,V)

Vector_rsw=zeros(3,1);

e_r=R/norm(R);
h=cross(R,V);
e_w=h/norm(h);
e_s=cross(e_w,e_r);


Vector_rsw(1)=dot(Vector_xyz,e_r);
Vector_rsw(2)=dot(Vector_xyz,e_s);
Vector_rsw(3)=dot(Vector_xyz,e_w);

end
